simulink model "RobotX_ss_acousticsSingle_Dock_LB_1024"  (R2014a)
settings: Solver=FixedStepDiscrete  StartTime=0.0  StopTime=inf  FixedStep=.25  RelTol=1e-3
undefined symbols (not defined in the file): Com1, Com2, Com3, Com4, DiscIntNeverNeededParam, standard
libraries: xpcseriallib x42, simulink x16, slrtlib x7, dspmtrx3 x2, speedgoatlib x2, speedgoatlib_IO102 x1
(part 3 of 6)

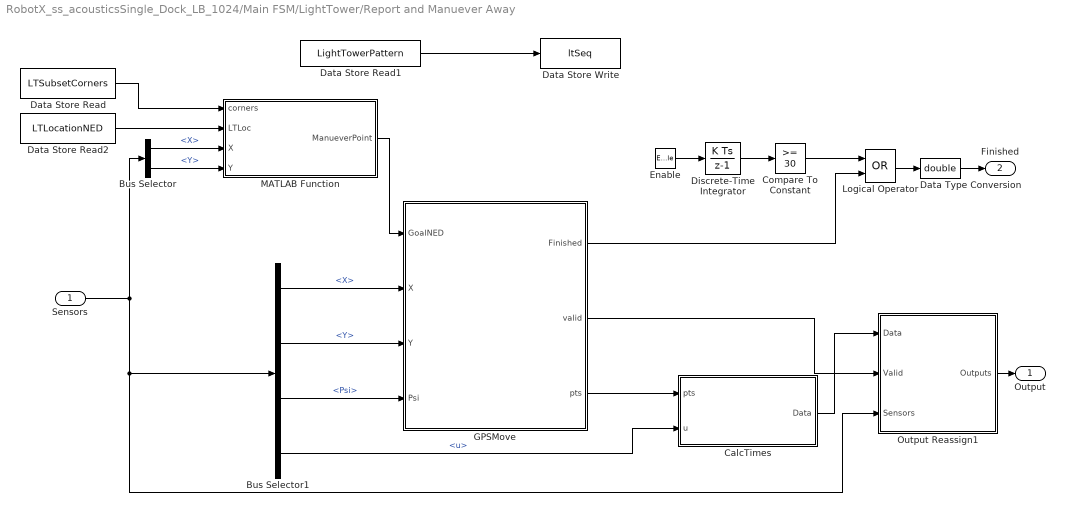
== system RobotX_ss_acousticsSingle_Dock_LB_1024/Main FSM/LightTower/Report and Manuever Away ==
  Sensors : Inport
  Enable : EnablePort  ShowOutputPort=on
  Bus Selector : BusSelector  OutputSignals=Navigation Message.Pose.X,Navigation Message.Pose.Y
  Bus Selector1 : BusSelector  OutputSignals=Navigation Message.Pose.X,Navigation Message.Pose.Y,Navigation Message.Pose.Psi,Navigation Message.Velocity.u
  CalcTimes : MATLAB Function  TreatAsAtomicUnit=on
  Compare To Constant : simulink/Logic and Bit Operations/Compare To Constant  relop=>=  const=30  OutDataTypeStr=boolean
  Data Store Read : DataStoreRead  DataStoreName=LTSubsetCorners
  Data Store Read1 : DataStoreRead  DialogController=Simulink.DDGSource  DataStoreName=LightTowerPattern
  Data Store Read2 : DataStoreRead  DialogController=Simulink.DDGSource  DataStoreName=LTLocationNED
  Data Store Write : DataStoreWrite  DialogController=Simulink.DDGSource  DataStoreName=ltSeq
  Data Type Conversion : DataTypeConversion  OutDataTypeStr=double
  Discrete-Time Integrator : DiscreteIntegrator  SampleTime=-1  ICPrevOutput=DiscIntNeverNeededParam  ICPrevScaledInput=DiscIntNeverNeededParam
  GPSMove : MATLAB Function  TreatAsAtomicUnit=on
  Logical Operator : Logic  Operator=OR  AllPortsSameDT=off  OutDataTypeStr=boolean
  MATLAB Function : MATLAB Function  TreatAsAtomicUnit=on
  Output Reassign1 : Subsystem
  Output : Outport
  Finished : Outport  Port=2
  wires:
  Output Reassign1/1(Outputs) -> Output/1
  Data Store Read/1 -> MATLAB Function/1(corners)
  Sensors/1 -> Bus Selector/1, Output Reassign1/3(Sensors), Bus Selector1/1
  Bus Selector/1 -> MATLAB Function/3(X)  "<X>"
  Bus Selector/2 -> MATLAB Function/4(Y)  "<Y>"
  GPSMove/1(Finished) -> Logical Operator/2
  GPSMove/3(pts) -> CalcTimes/1(pts)
  Bus Selector1/1 -> GPSMove/2(X)  "<X>"
  Bus Selector1/2 -> GPSMove/3(Y)  "<Y>"
  Bus Selector1/3 -> GPSMove/4(Psi)  "<Psi>"
  Bus Selector1/4 -> CalcTimes/2(u)  "<u>"
  CalcTimes/1(Data) -> Output Reassign1/1(Data)
  GPSMove/2(valid) -> Output Reassign1/2(Valid)
  MATLAB Function/1(ManueverPoint) -> GPSMove/1(GoalNED)
  Data Store Read1/1 -> Data Store Write/1
  Data Store Read2/1 -> MATLAB Function/2(LTLoc)
  Discrete-Time Integrator/1 -> Compare To Constant/1
  Enable/1 -> Discrete-Time Integrator/1
  Compare To Constant/1 -> Logical Operator/1
  Logical Operator/1 -> Data Type Conversion/1
  Data Type Conversion/1 -> Finished/1

== system RobotX_ss_acousticsSingle_Dock_LB_1024/Main FSM/LightTower/Sweep Field ==
  Sensors : Inport
  Enable : EnablePort  ShowOutputPort=on
  Bus Creator : BusCreator  Inputs=2
  Bus Selector : BusSelector  OutputSignals=Drive to Point Fin,Spin & Listen Fin
  Compare To Constant : simulink/Logic and Bit Operations/Compare To Constant  relop=>=  const=30  OutDataTypeStr=boolean
  Data Type Conversion : DataTypeConversion  OutDataTypeStr=double
  Discrete-Time Integrator : DiscreteIntegrator  SampleTime=-1  ICPrevOutput=DiscIntNeverNeededParam  ICPrevScaledInput=DiscIntNeverNeededParam
  Drive to Point : Subsystem
  Logical Operator : Logic  Operator=OR  Inputs=3  AllPortsSameDT=off  OutDataTypeStr=boolean
  Multiport Switch : MultiPortSwitch  Inputs=2
  "Spin, Listen, and Point" : Subsystem
  Sweep Field Enabler : MATLAB Function  TreatAsAtomicUnit=on
  Task Option : Subsystem
  Unit Delay : UnitDelay  SampleTime=-1
  Outputs : Outport
  Finished : Outport  Port=2
  wires:
  Drive to Point/1(Outputs) -> Multiport Switch/2
  "Spin, Listen, and Point"/1(Outputs) -> Multiport Switch/3
  Multiport Switch/1 -> Outputs/1
  Data Type Conversion/1 -> Finished/1
  Sensors/1 -> "Spin, Listen, and Point"/1(Sensors), Drive to Point/1(Sensors)
  Task Option/1(Option) -> Sweep Field Enabler/1(Sweep)
  "Spin, Listen, and Point"/2(Finished) -> Bus Creator/2  "Spin & Listen Fin"
  Sweep Field Enabler/2(drivePointEn) -> Drive to Point/Enable
  Sweep Field Enabler/1(taskSelector) -> Multiport Switch/1
  Sweep Field Enabler/3(spinListenEn) -> "Spin, Listen, and Point"/Enable
  Drive to Point/2(Finished) -> Bus Creator/1  "Drive to Point Fin"
  Bus Creator/1 -> Unit Delay/1
  "Spin, Listen, and Point"/3(Found LT) -> Logical Operator/2
  Unit Delay/1 -> Bus Selector/1
  Bus Selector/1 -> Sweep Field Enabler/2(drivePointFin)  "<Drive to Point Fin>"
  Bus Selector/2 -> Sweep Field Enabler/3(spinFin)  "<Spin & Listen Fin>"
  Drive to Point/3(Found LT) -> Logical Operator/1
  Logical Operator/1 -> Data Type Conversion/1
  Discrete-Time Integrator/1 -> Compare To Constant/1
  Enable/1 -> Discrete-Time Integrator/1
  Compare To Constant/1 -> Logical Operator/3

== system RobotX_ss_acousticsSingle_Dock_LB_1024/Main FSM/LightTower/Turn For Approach1  ==
  note: Signal
  Sensors : Inport
  Enable : EnablePort  ShowOutputPort=on
  Bus Selector : BusSelector  OutputSignals=Navigation Message.Pose.X,Navigation Message.Pose.Y
  Compare To Constant : simulink/Logic and Bit Operations/Compare To Constant  relop=>=  const=30  OutDataTypeStr=boolean
  Data Type Conversion : DataTypeConversion  OutDataTypeStr=double
  Discrete-Time Integrator : DiscreteIntegrator  SampleTime=-1  ICPrevOutput=DiscIntNeverNeededParam  ICPrevScaledInput=DiscIntNeverNeededParam
  LTLoc : DataStoreRead  DialogController=Simulink.DDGSource  DataStoreName=LTLocationNED
  MATLAB1 Function : MATLAB Function  TreatAsAtomicUnit=on
  Output Heirarchy : Subsystem
  Outputs : Outport
  Finished : Outport  Port=2
  wires:
  Discrete-Time Integrator/1 -> Compare To Constant/1
  Enable/1 -> Discrete-Time Integrator/1
  Compare To Constant/1 -> Data Type Conversion/1
  Data Type Conversion/1 -> Finished/1
  Sensors/1 -> Bus Selector/1, Output Heirarchy/2(Sensors)
  MATLAB1 Function/1(Data) -> Output Heirarchy/1(Data)
  Output Heirarchy/1(Outputs) -> Outputs/1
  Bus Selector/2 -> MATLAB1 Function/3(Y)  "<Y>"
  Bus Selector/1 -> MATLAB1 Function/2(X)  "<X>"
  LTLoc/1 -> MATLAB1 Function/1(LTLoc)

== system RobotX_ss_acousticsSingle_Dock_LB_1024/Main FSM/LightTower/Turn For Sweep ==
  note: Signal
  Sensors : Inport
  Enable : EnablePort  ShowOutputPort=on
  Bus Selector : BusSelector  OutputSignals=Navigation Message.Pose.X,Navigation Message.Pose.Y
  Compare To Constant : simulink/Logic and Bit Operations/Compare To Constant  relop=>=  const=30  OutDataTypeStr=boolean
  Data Store Read : DataStoreRead  DataStoreName=ltGPS
  Data Store Read1 : DataStoreRead  DataStoreName=NED_origin
  Data Type Conversion : DataTypeConversion  OutDataTypeStr=double
  Discrete-Time Integrator : DiscreteIntegrator  SampleTime=-1  ICPrevOutput=DiscIntNeverNeededParam  ICPrevScaledInput=DiscIntNeverNeededParam
  LLA to NED : MATLAB Function  TreatAsAtomicUnit=on
  MATLAB Function : MATLAB Function  TreatAsAtomicUnit=on
  Output Heirarchy : Subsystem
  Outputs : Outport
  Finished : Outport  Port=2
  wires:
  Discrete-Time Integrator/1 -> Compare To Constant/1
  Enable/1 -> Discrete-Time Integrator/1
  Compare To Constant/1 -> Data Type Conversion/1
  Data Type Conversion/1 -> Finished/1
  Sensors/1 -> Bus Selector/1, Output Heirarchy/2(Sensors)
  MATLAB Function/1(Data) -> Output Heirarchy/1(Data)
  Output Heirarchy/1(Outputs) -> Outputs/1
  Bus Selector/2 -> MATLAB Function/3(Y)  "<Y>"
  Bus Selector/1 -> MATLAB Function/2(X)  "<X>"
  Data Store Read/1 -> LLA to NED/1(GoalLLA)
  Data Store Read1/1 -> LLA to NED/2(NED_origin)
  LLA to NED/1(GoalNED) -> MATLAB Function/1(ltPTS)

== system RobotX_ss_acousticsSingle_Dock_LB_1024/Main FSM/LightTower/Wait for Sequence ==
  Sensors : Inport
  Enable : EnablePort  ShowOutputPort=on
  Bus Selector1 : BusSelector  OutputSignals=Lidar Data Input.Color data.Color
  Data Store Read : DataStoreRead  DataStoreName=holdPose
  Data Store Write : DataStoreWrite  DataStoreName=LightTowerPattern
  Discrete-Time Integrator : DiscreteIntegrator  SampleTime=-1  ICPrevOutput=DiscIntNeverNeededParam  ICPrevScaledInput=DiscIntNeverNeededParam
  MATLAB Function : MATLAB Function  TreatAsAtomicUnit=on
  MATLAB Function1 : MATLAB Function  TreatAsAtomicUnit=on
  Output Reassign1 : Subsystem
  Output : Outport
  Finished : Outport  Port=2
  wires:
  Sensors/1 -> Bus Selector1/1, Output Reassign1/2(Sensors)
  Output Reassign1/1(Outputs) -> Output/1
  MATLAB Function/1(Data) -> Output Reassign1/1(Data)
  MATLAB Function1/2(Pattern) -> Data Store Write/1
  Bus Selector1/1 -> MATLAB Function1/2(visionData)  "<Color>"
  Enable/1 -> Discrete-Time Integrator/1
  Discrete-Time Integrator/1 -> MATLAB Function1/1(time)
  MATLAB Function1/1(Finished) -> Finished/1
  Data Store Read/1 -> MATLAB Function/1(holdPose)

== system RobotX_ss_acousticsSingle_Dock_LB_1024/Main FSM/RCHold/Direct Control ==
  Sensors : Inport
  Acoustic Active : Constant  Value=0
  Bus Creator2 : BusCreator  Inputs=3
  Bus Creator3 : BusCreator  Inputs=3
  Bus Creator4 : BusCreator  Inputs=2
  Constant : Constant
  Constant1 : Constant  Value=2
  Constant2 : Constant  Value=zeros(24,1)
  Lidar Mode : Constant  Value=3
  Outputs : Outport
  wires:
  Sensors/1 -> Bus Creator4/2  "Sensors"
  Bus Creator4/1 -> Outputs/1  "Output Signals"
  Bus Creator2/1 -> Bus Creator3/1  "Navigation Outputs"
  Acoustic Active/1 -> Bus Creator3/2  "Acoustic Active"
  Lidar Mode/1 -> Bus Creator3/3  "Lidar Mode"
  Bus Creator3/1 -> Bus Creator4/1  "Outputs"
  Constant/1 -> Bus Creator2/1  "Valid"
  Constant1/1 -> Bus Creator2/2  "Control Mode"
  Constant2/1 -> Bus Creator2/3  "Data"

== system RobotX_ss_acousticsSingle_Dock_LB_1024/Main FSM/Start//Speedgate/Aim ==
  note: Signal
  Sensors : Inport
  Enable : EnablePort  ShowOutputPort=on
  Compare To Constant : simulink/Logic and Bit Operations/Compare To Constant  relop=>=  const=30  OutDataTypeStr=boolean
  Data Store Read : DataStoreRead  DataStoreName=ssHeldHeading
  Data Store Read1 : DataStoreRead  Commented=on  DataStoreName=startGPS
  Data Store Read2 : DataStoreRead  Commented=on  DataStoreName=NED_origin
  Data Store Read3 : DataStoreRead  DataStoreName=startNED
  Data Type Conversion : DataTypeConversion  OutDataTypeStr=double
  Discrete-Time Integrator : DiscreteIntegrator  SampleTime=-1  ICPrevOutput=DiscIntNeverNeededParam  ICPrevScaledInput=DiscIntNeverNeededParam
  LLA to NED : MATLAB Function  Commented=on  TreatAsAtomicUnit=on
  MATLAB Function : MATLAB Function  TreatAsAtomicUnit=on
  Output Heirarchy : Subsystem
  Outputs : Outport
  Finished : Outport  Port=2
  wires:
  Discrete-Time Integrator/1 -> Compare To Constant/1
  Enable/1 -> Discrete-Time Integrator/1
  Compare To Constant/1 -> Data Type Conversion/1
  Data Type Conversion/1 -> Finished/1
  Sensors/1 -> Output Heirarchy/2(Sensors)
  MATLAB Function/1(Data) -> Output Heirarchy/1(Data)
  Output Heirarchy/1(Outputs) -> Outputs/1
  Data Store Read/1 -> MATLAB Function/1(ssHeldHeading)
  LLA to NED/1(GoalNED) -> ?
  Data Store Read2/1 -> LLA to NED/2(NED_origin)
  Data Store Read1/1 -> LLA to NED/1(LLA)
  Data Store Read3/1 -> MATLAB Function/2(ssGateNED)

== system RobotX_ss_acousticsSingle_Dock_LB_1024/Main FSM/Start//Speedgate/Dead Reckon ==
  note: Through Gate
  Sensors : Inport
  Enable : EnablePort
  Bus Selector : BusSelector  OutputSignals=Navigation Message.Pose.X,Navigation Message.Pose.Y,Navigation Message.Velocity.u
  Calculate Times : MATLAB Function  TreatAsAtomicUnit=on
  Data Store Read : DataStoreRead  DataStoreName=ssHeldHeading
  Gate : MATLAB Function  TreatAsAtomicUnit=on
  Output Reassign : Subsystem
  sglength : Constant  Value=15
  Outputs : Outport
  Finished : Outport  Port=2
  wires:
  Output Reassign/1(Outputs) -> Outputs/1
  Gate/1(Finished) -> Finished/1
  Sensors/1 -> Output Reassign/3(Sensors), Bus Selector/1
  Bus Selector/2 -> Gate/4(Y)  "<Y>"
  Bus Selector/1 -> Gate/3(X)  "<X>"
  Bus Selector/3 -> Calculate Times/2(u)  "<u>"
  Gate/3(pts) -> Calculate Times/1(pts)
  Calculate Times/1(Data) -> Output Reassign/2(Data)
  Gate/2(Valid) -> Output Reassign/1(Vaild)
  Data Store Read/1 -> Gate/2(ssHeldHeading)
  sglength/1 -> Gate/1(sglength)

== system RobotX_ss_acousticsSingle_Dock_LB_1024/Main FSM/Start//Speedgate/GPS Move ==
  Sensors : Inport
  Enable : EnablePort
  Bus Selector : BusSelector  OutputSignals=Navigation Message.Pose.X,Navigation Message.Pose.Y,Navigation Message.Pose.Psi,Navigation Message.Velocity.u
  CalcTimes : MATLAB Function  TreatAsAtomicUnit=on
  Data Store Read1 : DataStoreRead  Commented=on  DataStoreName=startGPS
  Data Store Read2 : DataStoreRead  Commented=on  DataStoreName=NED_origin
  Data Store Read3 : DataStoreRead  DataStoreName=startNED
  GPSMove : MATLAB Function  TreatAsAtomicUnit=on
  LLA to NED : MATLAB Function  Commented=on  TreatAsAtomicUnit=on
  Output Reassign : Subsystem
  Outputs : Outport
  Finished : Outport  Port=2
  wires:
  GPSMove/3(pts) -> CalcTimes/1(pts)
  Sensors/1 -> Output Reassign/3(Sensors), Bus Selector/1
  Bus Selector/1 -> GPSMove/2(X)  "<X>"
  Bus Selector/2 -> GPSMove/3(Y)  "<Y>"
  Bus Selector/3 -> GPSMove/4(Psi)  "<Psi>"
  Bus Selector/4 -> CalcTimes/2(u)  "<u>"
  GPSMove/1(Finished) -> Finished/1
  Output Reassign/1(Outputs) -> Outputs/1
  CalcTimes/1(Data) -> Output Reassign/2(Data)
  GPSMove/2(valid) -> Output Reassign/1(Vaild)
  LLA to NED/1(GoalNED) -> ?
  Data Store Read3/1 -> GPSMove/1(GoalNED)
  Data Store Read2/1 -> LLA to NED/2(NED_origin)
  Data Store Read1/1 -> LLA to NED/1(LLA)

== system RobotX_ss_acousticsSingle_Dock_LB_1024/Main FSM/Termination/Output Reassign ==
  Vaild : Inport
  Data : Inport  Port=2
  Sensors : Inport  Port=3
  Acoustic Active : Constant  Value=0
  Bus Creator2 : BusCreator  Inputs=3
  Bus Creator3 : BusCreator  Inputs=3
  Bus Creator5 : BusCreator  Inputs=2
  Constant3 : Constant  Value=0
  Lidar Mode : Constant  Value=0
  Outputs : Outport
  wires:
  Sensors/1 -> Bus Creator5/2  "Sensors"
  Bus Creator5/1 -> Outputs/1  "Output Signals"
  Vaild/1 -> Bus Creator2/1  "Valid"
  Constant3/1 -> Bus Creator2/2  "Control Mode"
  Data/1 -> Bus Creator2/3  "Data"
  Bus Creator2/1 -> Bus Creator3/1  "Navigation Outputs"
  Acoustic Active/1 -> Bus Creator3/2  "Acoustic Active"
  Lidar Mode/1 -> Bus Creator3/3  "Lidar Mode"
  Bus Creator3/1 -> Bus Creator5/1  "Outputs"

== system RobotX_ss_acousticsSingle_Dock_LB_1024/Sensors/1020 Comms/ Raspberry Pi LCM (Acoustic) ==
  LCM Input : Inport
  ASCII Decode 6 : xpcseriallib/ASCII Decode   format=Deploy:%1u, Elapsed:%g, Bearing1:%g Bearing2:%g \r\n  nvars=4  vartypes={}
  Bus Creator : BusCreator  Inputs=2
  Bus Creator1 : BusCreator  Inputs=3
  FIFO ASCII read 1 : xpcseriallib/FIFO ASCII read   header={'Deploy:'}  term=[13 10]  hold=Zero output if no new data  enable=off  maxsize=1024  outputtype=8 bit uint null terminated  sampletime=-1
  LCM Output : Outport
  wires:
  LCM Input/1 -> FIFO ASCII read 1/1
  FIFO ASCII read 1/1 -> ASCII Decode 6/1
  ASCII Decode 6/3 -> Bus Creator/1  "Horizontal Bearing"
  ASCII Decode 6/4 -> Bus Creator/2  "Vertical Bearing"
  Bus Creator/1 -> Bus Creator1/3  "Bearings"
  ASCII Decode 6/2 -> Bus Creator1/2  "Elapsed Time"
  ASCII Decode 6/1 -> Bus Creator1/1  "Deployed"
  Bus Creator1/1 -> LCM Output/1  "Acoustic Message"

== system RobotX_ss_acousticsSingle_Dock_LB_1024/Sensors/1020 Comms/ Raspberry Pi LCM (Navigation and Acoustics) ==
  LCM Input : Inport
  ASCII Decode 6 : xpcseriallib/ASCII Decode   format=P1:%f P2:%f P3:%f V1:%f V2:%f V3:%f E1:%f E2:%f E3:%f Pt1:%f Pt2:%f St1:%f St2:%f Start:%f Elapsed:%f RC:%d Deploy:%u, Elapsed:%g, Bearing1:%g Bearing2:%g \r\n  nvars=22  vartypes={}
  Bus Creator{,5..7} (4 alike) : BusCreator  Inputs=2
  Bus Creator{1..3,8} (4 alike) : BusCreator  Inputs=3
  Bus Creator4 : BusCreator  Inputs=9
  Data Type Conversion : DataTypeConversion  OutDataTypeStr=double
  FIFO ASCII read 1 : xpcseriallib/FIFO ASCII read   header={'P1:'}  term=[13 10]  hold=Zero output if no new data  enable=off  maxsize=2048  outputtype=8 bit uint null terminated  sampletime=-1
  Navigation LCM : Outport
  Acoustic LCM : Outport  Port=2
  wires:
  LCM Input/1 -> FIFO ASCII read 1/1
  FIFO ASCII read 1/1 -> ASCII Decode 6/1
  Bus Creator4/1 -> Navigation LCM/1  "Navigation Message"
  ASCII Decode 6/1 -> Bus Creator1/1  "X"
  ASCII Decode 6/2 -> Bus Creator1/2  "Y"
  ASCII Decode 6/3 -> Bus Creator1/3  "Psi"
  Bus Creator1/1 -> Bus Creator4/1  "Pose"
  ASCII Decode 6/4 -> Bus Creator2/1  "u"
  ASCII Decode 6/5 -> Bus Creator2/2  "v"
  Bus Creator2/1 -> Bus Creator4/2  "Velocity"
  ASCII Decode 6/7 -> Bus Creator3/1  "Roll"
  ASCII Decode 6/8 -> Bus Creator3/2  "Pitch"
  ASCII Decode 6/9 -> Bus Creator3/3  "Yaw"
  Bus Creator3/1 -> Bus Creator4/3  "Euler"
  Bus Creator5/1 -> Bus Creator4/5  "Port"
  Bus Creator6/1 -> Bus Creator4/6  "Stbd"
  ASCII Decode 6/14 -> Bus Creator6/1  "StThrust"
  ASCII Decode 6/15 -> Bus Creator6/2  "StAzimuth"
  ASCII Decode 6/12 -> Bus Creator5/1  "PtThrust"
  ASCII Decode 6/13 -> Bus Creator5/2  "PtAzimuth"
  ASCII Decode 6/16 -> Bus Creator4/7  "Start"
  ASCII Decode 6/17 -> Bus Creator4/8  "Elapsed"
  ASCII Decode 6/18 -> Data Type Conversion/1  "On/Off/RC/Auto"
  Data Type Conversion/1 -> Bus Creator4/9  "On/Off/RC/Auto"
  ASCII Decode 6/6 -> Bus Creator2/3  "r"
  ASCII Decode 6/10 -> Bus Creator7/1  "Lat"
  ASCII Decode 6/11 -> Bus Creator7/2  "Long"
  Bus Creator7/1 -> Bus Creator4/4  "GPS (LLA)"
  ASCII Decode 6/21 -> Bus Creator/1  "Horizontal Bearing"
  ASCII Decode 6/22 -> Bus Creator/2  "Vertical Bearing"
  Bus Creator/1 -> Bus Creator8/3  "Bearings"
  ASCII Decode 6/20 -> Bus Creator8/2  "Elapsed Time"
  ASCII Decode 6/19 -> Bus Creator8/1  "Deployed"
  Bus Creator8/1 -> Acoustic LCM/1  "Acoustic Message"

== system RobotX_ss_acousticsSingle_Dock_LB_1024/Sensors/1020 Comms/ Raspberry Pi LCM (Navigation) ==
  LCM Input : Inport
  ASCII Decode 6 : xpcseriallib/ASCII Decode   format=P1:%f P2:%f P3:%f V1:%f V2:%f V3:%f E1:%f E2:%f E3:%f Lat:%f Long:%f Pt1:%f Pt2:%f St1:%f St2:%f Start:%f Elapsed:%f RC:%d Deploy:%u Elapsed:%f Bearing1:%f Bearing2:%f Range:%f X_Pos:%f Y_Pos:%f \r\n  nvars=25  vartypes={}
  Bus Creator1 : BusCreator  Inputs=3
  Bus Creator2 : BusCreator  Inputs=3
  Bus Creator3 : BusCreator  Inputs=3
  Bus Creator4 : BusCreator  Inputs=9
  Bus Creator5 : BusCreator  Inputs=2
  Bus Creator6 : BusCreator  Inputs=2
  Bus Creator7 : BusCreator  Inputs=2
  Bus Creator8 : BusCreator  Inputs=7
  Data Type Conversion : DataTypeConversion  OutDataTypeStr=double
  FIFO ASCII read 1 : xpcseriallib/FIFO ASCII read   header={'P1:'}  term=[13 10]  hold=Zero output if no new data  enable=off  maxsize=2000  outputtype=8 bit uint null terminated  sampletime=-1
  LCM Output : Outport
  Acou LCM : Outport  Port=2
  wires:
  LCM Input/1 -> FIFO ASCII read 1/1
  FIFO ASCII read 1/1 -> ASCII Decode 6/1
  Bus Creator4/1 -> LCM Output/1  "Navigation Message"
  ASCII Decode 6/1 -> Bus Creator1/1  "X"
  ASCII Decode 6/2 -> Bus Creator1/2  "Y"
  ASCII Decode 6/3 -> Bus Creator1/3  "Psi"
  Bus Creator1/1 -> Bus Creator4/1  "Pose"
  ASCII Decode 6/4 -> Bus Creator2/1  "u"
  ASCII Decode 6/5 -> Bus Creator2/2  "v"
  Bus Creator2/1 -> Bus Creator4/2  "Velocity"
  ASCII Decode 6/7 -> Bus Creator3/1  "Roll"
  ASCII Decode 6/8 -> Bus Creator3/2  "Pitch"
  ASCII Decode 6/9 -> Bus Creator3/3  "Yaw"
  Bus Creator3/1 -> Bus Creator4/3  "Euler"
  Bus Creator5/1 -> Bus Creator4/5  "Port"
  Bus Creator6/1 -> Bus Creator4/6  "Stbd"
  ASCII Decode 6/14 -> Bus Creator6/1  "StThrust"
  ASCII Decode 6/15 -> Bus Creator6/2  "StAzimuth"
  ASCII Decode 6/12 -> Bus Creator5/1  "PtThrust"
  ASCII Decode 6/13 -> Bus Creator5/2  "PtAzimuth"
  ASCII Decode 6/16 -> Bus Creator4/7  "Start"
  ASCII Decode 6/17 -> Bus Creator4/8  "Elapsed"
  ASCII Decode 6/18 -> Data Type Conversion/1  "On/Off/RC/Auto"
  Data Type Conversion/1 -> Bus Creator4/9  "On/Off/RC/Auto"
  ASCII Decode 6/6 -> Bus Creator2/3  "r"
  ASCII Decode 6/10 -> Bus Creator7/1  "Lat"
  ASCII Decode 6/11 -> Bus Creator7/2  "Long"
  Bus Creator7/1 -> Bus Creator4/4  "GPS (LLA)"
  ASCII Decode 6/19 -> Bus Creator8/1  "Deployed"
  ASCII Decode 6/20 -> Bus Creator8/2  "Elapsed Time"
  ASCII Decode 6/21 -> Bus Creator8/3  "Horizontal Bearing"
  ASCII Decode 6/22 -> Bus Creator8/4  "Vertical Bearing"
  ASCII Decode 6/23 -> Bus Creator8/5  "Range"
  ASCII Decode 6/24 -> Bus Creator8/6  "X Pos"
  ASCII Decode 6/25 -> Bus Creator8/7  "Y Pos"
  Bus Creator8/1 -> Acou LCM/1

== system RobotX_ss_acousticsSingle_Dock_LB_1024/Sensors/1020 Comms/Acoustic LCM ==
  LCM Input : Inport
  Bus Creator : BusCreator  Inputs=2
  Bus Creator1 : BusCreator
  Bus Creator2 : BusCreator  Inputs=3
  Bus Selector : BusSelector  OutputSignals=Deployed,Elapsed Time,Horizontal Bearing,Vertical Bearing,Range,X Pos,Y Pos
  LCM Output : Outport
  wires:
  Bus Selector/3 -> Bus Creator/1  "<Horizontal Bearing>"
  Bus Selector/4 -> Bus Creator/2  "<Vertical Bearing>"
  Bus Creator/1 -> Bus Creator1/3  "Bearings"
  Bus Selector/2 -> Bus Creator1/2  "<Elapsed Time>"
  Bus Selector/1 -> Bus Creator1/1  "<Deployed>"
  Bus Creator1/1 -> LCM Output/1  "Acoustic Message"
  LCM Input/1 -> Bus Selector/1
  Bus Selector/5 -> Bus Creator2/1  "<Range>"
  Bus Selector/6 -> Bus Creator2/2  "<X Pos>"
  Bus Selector/7 -> Bus Creator2/3  "<Y Pos>"
  Bus Creator2/1 -> Bus Creator1/4  "Pose Estimate"

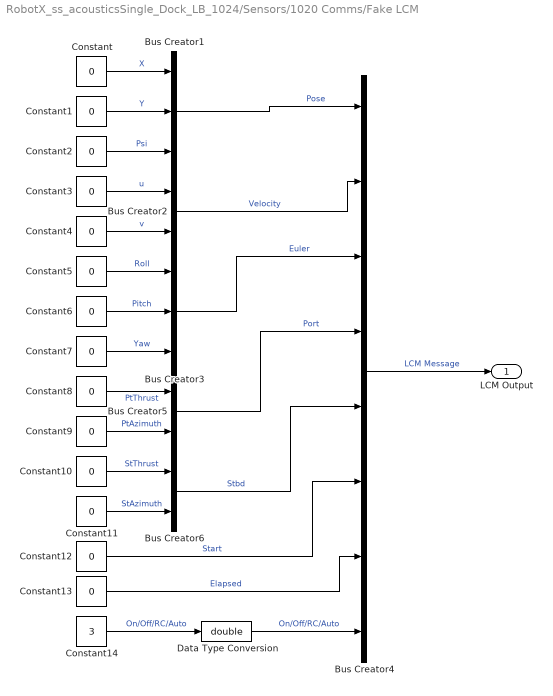
== system RobotX_ss_acousticsSingle_Dock_LB_1024/Sensors/1020 Comms/Fake LCM ==
  Bus Creator1 : BusCreator  Inputs=3
  Bus Creator2 : BusCreator  Inputs=2
  Bus Creator3 : BusCreator  Inputs=3
  Bus Creator4 : BusCreator  Inputs=8
  Bus Creator5 : BusCreator  Inputs=2
  Bus Creator6 : BusCreator  Inputs=2
  Constant{,1..13} (14 alike) : Constant  Value=0
  Constant14 : Constant  Value=3
  Data Type Conversion : DataTypeConversion  OutDataTypeStr=double
  LCM Output : Outport
  wires:
  Bus Creator4/1 -> LCM Output/1  "LCM Message"
  Constant/1 -> Bus Creator1/1  "X"
  Constant1/1 -> Bus Creator1/2  "Y"
  Constant2/1 -> Bus Creator1/3  "Psi"
  Bus Creator1/1 -> Bus Creator4/1  "Pose"
  Constant3/1 -> Bus Creator2/1  "u"
  Constant4/1 -> Bus Creator2/2  "v"
  Bus Creator2/1 -> Bus Creator4/2  "Velocity"
  Constant5/1 -> Bus Creator3/1  "Roll"
  Constant6/1 -> Bus Creator3/2  "Pitch"
  Constant7/1 -> Bus Creator3/3  "Yaw"
  Bus Creator3/1 -> Bus Creator4/3  "Euler"
  Bus Creator5/1 -> Bus Creator4/4  "Port"
  Bus Creator6/1 -> Bus Creator4/5  "Stbd"
  Constant10/1 -> Bus Creator6/1  "StThrust"
  Constant11/1 -> Bus Creator6/2  "StAzimuth"
  Constant8/1 -> Bus Creator5/1  "PtThrust"
  Constant9/1 -> Bus Creator5/2  "PtAzimuth"
  Constant12/1 -> Bus Creator4/6  "Start"
  Constant13/1 -> Bus Creator4/7  "Elapsed"
  Constant14/1 -> Data Type Conversion/1  "On/Off/RC/Auto"
  Data Type Conversion/1 -> Bus Creator4/8  "On/Off/RC/Auto"

== system RobotX_ss_acousticsSingle_Dock_LB_1024/Sensors/1020 Comms/LIDAR Panda ==
  LIDAR Panda In : Inport
  ASCII Decode 2 : xpcseriallib/ASCII Decode   format=A:%d B:%d C:%d E:%d F:%d G:%d H:%d I:%d J:%d K:%d L:%d M:%d N:%d O:%d P:%d Q:%d R:%d S:%d T:%d U:%d V:%d W:%d X:%d C1:%d C2:%d C3:%d C4:%d P1:%f P2:%f P3:%f P4:%f I1:%d I2:%d I3:%d I4:%d \r\n  nvars=36  vartypes={}
  Bus Creator1 : BusCreator  Inputs=2
  Bus Creator2 : BusCreator  Inputs=3
  Bus Creator3 : BusCreator  Inputs=2
  Data Type Conversion{,1..3} (4 alike) : DataTypeConversion  OutDataTypeStr=double
  "FIFO ASCII read " : xpcseriallib/FIFO ASCII read   header={'A:'}  term=[13 10]  hold=Zero output if no new data  enable=off  maxsize=1024  outputtype=8 bit uint null terminated  sampletime=-1
  Mux : Mux  Inputs=12
  Mux1 : Mux
  Mux2 : Mux  Inputs=12
  Mux3 : Mux
  Mux4 : Mux
  LIDAR Panda Out : Outport
  wires:
  LIDAR Panda In/1 -> "FIFO ASCII read "/1
  "FIFO ASCII read "/1 -> ASCII Decode 2/1
  ASCII Decode 2/3 -> Mux/3  "Distance"
  ASCII Decode 2/2 -> Mux/2  "Color ID"
  ASCII Decode 2/4 -> Mux/4  "Angle"
  ASCII Decode 2/1 -> Mux/1  "Probability"
  ASCII Decode 2/7 -> Mux/7
  ASCII Decode 2/10 -> Mux/10
  ASCII Decode 2/11 -> Mux/11
  ASCII Decode 2/6 -> Mux/6
  ASCII Decode 2/8 -> Mux/8
  ASCII Decode 2/9 -> Mux/9
  ASCII Decode 2/12 -> Mux/12
  ASCII Decode 2/5 -> Mux/5
  ASCII Decode 2/13 -> Mux2/1
  ASCII Decode 2/15 -> Mux2/3
  ASCII Decode 2/22 -> Mux2/10
  ASCII Decode 2/23 -> Mux2/11
  ASCII Decode 2/17 -> Mux2/5
  ASCII Decode 2/18 -> Mux2/6
  ASCII Decode 2/14 -> Mux2/2
  ASCII Decode 2/24 -> Mux2/12
  ASCII Decode 2/20 -> Mux2/8
  ASCII Decode 2/19 -> Mux2/7
  ASCII Decode 2/21 -> Mux2/9
  ASCII Decode 2/16 -> Mux2/4
  ASCII Decode 2/25 -> Mux1/1
  ASCII Decode 2/28 -> Mux1/4
  ASCII Decode 2/26 -> Mux1/2
  ASCII Decode 2/27 -> Mux1/3
  ASCII Decode 2/30 -> Mux3/2
  ASCII Decode 2/31 -> Mux3/3
  ASCII Decode 2/32 -> Mux3/4
  ASCII Decode 2/29 -> Mux3/1
  ASCII Decode 2/36 -> Mux4/4
  ASCII Decode 2/34 -> Mux4/2
  ASCII Decode 2/35 -> Mux4/3
  ASCII Decode 2/33 -> Mux4/1
  Mux/1 -> Data Type Conversion/1  "Distances"
  Mux2/1 -> Data Type Conversion1/1  "Angles"
  Mux1/1 -> Data Type Conversion2/1  "Color"
  Mux3/1 -> Bus Creator2/2  "Probability"
  Mux4/1 -> Data Type Conversion3/1  "idx"
  Bus Creator1/1 -> Bus Creator3/1  "Landmarks"
  Bus Creator2/1 -> Bus Creator3/2  "Color data"
  Bus Creator3/1 -> LIDAR Panda Out/1
  Data Type Conversion/1 -> Bus Creator1/1  "Distances"
  Data Type Conversion1/1 -> Bus Creator1/2  "Angles"
  Data Type Conversion2/1 -> Bus Creator2/1  "Color"
  Data Type Conversion3/1 -> Bus Creator2/3  "Color"

== system RobotX_ss_acousticsSingle_Dock_LB_1024/Sensors/1020 Comms/Subsystem ==
  Bus Creator : BusCreator  Inputs=3
  Bus Creator1 : BusCreator  Inputs=2
  Bus Creator2 : BusCreator  Inputs=2
  Constant : Constant  Value=zeros(12,1)
  Constant1 : Constant  Value=zeros(12,1)
  Constant2 : Constant  Value=zeros(4,1)
  Constant3 : Constant  Value=zeros(4,1)
  Constant4 : Constant  Value=zeros(4,1)
  Fake Panda : Outport
  wires:
  Constant/1 -> Bus Creator1/1  "Distances"
  Constant1/1 -> Bus Creator1/2  "Angles"
  Constant2/1 -> Bus Creator/1  "Color"
  Constant3/1 -> Bus Creator/2  "Probability"
  Constant4/1 -> Bus Creator/3  "idx"
  Bus Creator1/1 -> Bus Creator2/1  "Landmarks"
  Bus Creator/1 -> Bus Creator2/2  "Color data"
  Bus Creator2/1 -> Fake Panda/1  "Lidar Data Input"

== system RobotX_ss_acousticsSingle_Dock_LB_1024/Sensors/1020 Comms/data log ==
  Sensors signal : Inport
  Bus Selector3 : BusSelector  OutputSignals=Navigation Message,Lidar Data Input,Acoustic Message
  Bus to Vector : BusToVector
  Bus to Vector1 : BusToVector
  Bus to Vector2 : BusToVector
  Read : DataStoreRead  DataStoreName=PingPose
  Scope 1 : slrtlib/Displays and Logging/Scope   scopeno=3  scopetype=File  autostart=on  viewmode=Graphical redraw  formatstr='%15.6f'  grid=on  ylimits=[0,0]  nosamples=28800  noprepostsamples=0  interleave=1  triggermode=FreeRun  triggersignal=1  trigsignalfromport=off  triggerlevel=0.0  triggerslope=Either  triggerscope=1  triggersample=0  filename=LM1_<%%%>.dat  mode=Lazy  writesize=5120  autorestart=on  dynamicfilemode=on  maxwritefilesize=512*1024^2
  Scope 2 : slrtlib/Displays and Logging/Scope   scopeno=1  scopetype=File  autostart=on  viewmode=Graphical redraw  formatstr='%15.6f'  grid=on  ylimits=[0,0]  nosamples=28800  noprepostsamples=0  interleave=1  triggermode=FreeRun  triggersignal=1  trigsignalfromport=off  triggerlevel=0.0  triggerslope=Either  triggerscope=1  triggersample=0  filename=NAV1_<%%%>.dat  mode=Lazy  writesize=5120  autorestart=on  dynamicfilemode=on  maxwritefilesize=512*1024^2
  Scope 3 : slrtlib/Displays and Logging/Scope   scopeno=2  scopetype=File  autostart=on  viewmode=Graphical redraw  formatstr='%15.6f'  grid=on  ylimits=[0,0]  nosamples=28800  noprepostsamples=0  interleave=1  triggermode=FreeRun  triggersignal=1  trigsignalfromport=off  triggerlevel=0.0  triggerslope=Either  triggerscope=1  triggersample=0  filename=ACO1_<%%%>.dat  mode=Lazy  writesize=5120  autorestart=on  dynamicfilemode=on  maxwritefilesize=512*1024^2
  Scope 4 : slrtlib/Displays and Logging/Scope   scopeno=4  scopetype=File  autostart=on  viewmode=Graphical redraw  formatstr='%15.6f'  grid=on  ylimits=[0,0]  nosamples=28800  noprepostsamples=0  interleave=1  triggermode=FreeRun  triggersignal=1  trigsignalfromport=off  triggerlevel=0.0  triggerslope=Either  triggerscope=1  triggersample=0  filename=pPos_<%%%>.dat  mode=Lazy  writesize=5120  autorestart=on  dynamicfilemode=on  maxwritefilesize=512*1024^2
  wires:
  Sensors signal/1 -> Bus Selector3/1
  Bus to Vector/1 -> Scope 2/1
  Bus Selector3/1 -> Bus to Vector/1  "<Navigation Message>"
  Bus to Vector1/1 -> Scope 1/1
  Bus to Vector2/1 -> Scope 3/1
  Bus Selector3/3 -> Bus to Vector2/1  "<Acoustic Message>"
  Bus Selector3/2 -> Bus to Vector1/1  "<Lidar Data Input>"
  Read/1 -> Scope 4/1

== system RobotX_ss_acousticsSingle_Dock_LB_1024/Sensors/1024 Comms/ Raspberry Pi LCM (Acoustic) ==
  LCM Input : Inport
  ASCII Decode 6 : xpcseriallib/ASCII Decode   format=Deploy:%1u, Elapsed:%g, Bearing1:%g Bearing2:%g \r\n  nvars=4  vartypes={}
  Bus Creator : BusCreator  Inputs=2
  Bus Creator1 : BusCreator  Inputs=3
  FIFO ASCII read 1 : xpcseriallib/FIFO ASCII read   header={'Deploy:'}  term=[13 10]  hold=Zero output if no new data  enable=off  maxsize=1024  outputtype=8 bit uint null terminated  sampletime=-1
  LCM Output : Outport
  wires:
  LCM Input/1 -> FIFO ASCII read 1/1
  FIFO ASCII read 1/1 -> ASCII Decode 6/1
  ASCII Decode 6/3 -> Bus Creator/1  "Horizontal Bearing"
  ASCII Decode 6/4 -> Bus Creator/2  "Vertical Bearing"
  Bus Creator/1 -> Bus Creator1/3  "Bearings"
  ASCII Decode 6/2 -> Bus Creator1/2  "Elapsed Time"
  ASCII Decode 6/1 -> Bus Creator1/1  "Deployed"
  Bus Creator1/1 -> LCM Output/1  "Acoustic Message"

== matlab function RobotX_ss_acousticsSingle_Dock_LB_1024/Sensors/1024 Comms/Message Selector/HRTLIT Message/MATLAB Function ==
  data: Time input; HRTLat input; HRTLong input; HRTTask input; HRTMode input; LITValid input; asciiHRTLIT output; LITSequence input
function asciiHRTLIT = asciiHRTLITEncoder(Time,HRTLat,HRTLong,HRTTask,HRTMode,LITValid,LITSequence)
% Initialize output message vector as the serial output block expects 128
% character message
asciiHRTLIT = uint8(zeros(1,128));

asciiComma = uint8(',');
asciiDeciPt = uint8('.');
asciiTeamID = uint8('FAUVU,');
asciiMsgEnd = uint8('*');
asciiMsgCRLF = [13 10];

% Convert UTC Time input (hhmmss) into ascii code
asciiTime = uint8(zeros(1,7));
asciiTime(7) = asciiComma;

for timeChar = 1:6
    asciiTime(timeChar) = floor(mod(Time,10^(7-timeChar))/...
        10^(6-timeChar)) + 48;
end

%%%%%%%%%%%%%%%%%%%%%%%%%%%%%%%%%%%%%%%%%%%%%%%%%%%%%%%%%%%%%%%%%%%%
% Heartbeat message
% Convert static strings to ascii code
asciiHRTMsgID = uint8('$RXHRT,');
if HRTLat >= 0
    asciiHRTNS = uint8('N,');
else
    HRTLat = -HRTLat;
    asciiHRTNS = uint8('S,');
end
if HRTLong >= 0
    asciiHRTEW = uint8('E,');
else
    HRTLong = -HRTLong;
    asciiHRTEW = uint8('W,');
end

% Convert latitude (dd.mmmmmm) into ascii code
asciiHRTLat = uint8(zeros(1,10));
asciiHRTLat(10) = asciiComma;
asciiHRTLat(3) = asciiDeciPt;

HRTlatInt = floor(HRTLat);
for latIntChar = 1:2
    asciiHRTLat(latIntChar) = floor(mod(HRTlatInt,10^(3-latIntChar))/...
        10^(2-latIntChar)) + 48;
end

HRTlatDeci = mod(HRTLat,HRTlatInt) * 10^6;
for latDeciChar = 1:6
    asciiHRTLat(latDeciChar+3) = floor(mod(HRTlatDeci,10^(7-latDeciChar))/...
        10^(6-latDeciChar)) + 48;
end

% Convert longitude (ddd.mmmmmm) into ascii code
asciiHRTLong = uint8(zeros(1,11));
asciiHRTLong(11) = asciiComma;
asciiHRTLong(4) = asciiDeciPt;

HRTlongInt = floor(HRTLong);
for longIntChar = 1:3
    asciiHRTLong(longIntChar) = floor(mod(HRTlongInt,10^(4-longIntChar))/...
        10^(3-longIntChar)) + 48;
end

HRTlongDeci = mod(HRTLong,HRTlongInt) * 10^6;
for longDeciChar = 1:6
    asciiHRTLong(longDeciChar+4) = floor(mod(HRTlongDeci,10^(7-longDeciChar))/...
        10^(6-longDeciChar)) + 48;
end

% Convert vehicle mode into ascii (1 = RC, 2 = Auto)

% Auto On 
if HRTMode == 3 
    HRTOpMode = 2;
    asciiHRTMode = [uint8(HRTOpMode+48) asciiComma];
else
    HRTOpMode = 1;
    asciiHRTMode = [uint8(HRTOpMode+48) asciiComma];
end

% Convert vehicle task into ascii
HRTTask = HRTTask - 1; % FSM: Init = 1, SSGate = 2, SEA = 3, Dock = 4, LIT = 5, Obst = 6
if HRTTask ~= 1 || 2 || 3 || 4 || 5
    HRTOpTask = 1;
    asciiHRTTask = [uint8(HRTOpTask+48) asciiMsgEnd];
else
    asciiHRTTask = [uint8(HRTTask+48) asciiMsgEnd];
end

% Concat individual ascii arrays into one array
asciiHRTPreChkSum = cat(2,asciiHRTMsgID,asciiTime,asciiHRTLat,asciiHRTNS,asciiHRTLong,asciiHRTEW,...
    asciiTeamID,asciiHRTMode,asciiHRTTask);

% Calculate the checksum of the message from the '$' to the '*' and convert
% to hex
HRTchkSum = uint8(0);

for chksumChar = 1:(length(asciiHRTPreChkSum)-2)
    HRTchkSum = bitxor(HRTchkSum,asciiHRTPreChkSum(chksumChar+1));
end

% Convert the checksum to ascii
HRTchkSum = dec2hex(HRTchkSum);
asciiHRTChkSum = uint8(zeros(1,length(HRTchkSum))+32);
for i = 1:length(HRTchkSum)
    asciiHRTChkSum(i) = uint8(HRTchkSum(i));
end

% Concat the checksum and the '/r/n' to the end of the message
asciiHRTPostChkSum = cat(2,asciiHRTPreChkSum,asciiHRTChkSum,asciiMsgCRLF);

%%%%%%%%%%%%%%%%%%%%%%%%%%%%%%%%%%%%%%%%%%%%%%%%%%%%%%%%%%%%%%%%%%%%%

% Light tower message
asciiLITMsgID = uint8('$RXLIT,');

% Convert the light sequece into ascii code (1 = R, 2 = B, 3 = G)
asciiLITSeq = uint8(zeros(1,4)+32);
asciiLITSeq(4) = asciiMsgEnd;

if LITValid == 1
    for seqChar = 1:3
        if LITSequence(seqChar) == 1
            LITSequence(seqChar) = uint8('R');
        elseif LITSequence(seqChar) == 2
            LITSequence(seqChar) = uint8('B');
        elseif LITSequence(seqChar) == 3
            LITSequence(seqChar) = uint8('G');
        end
    end
    asciiLITSeq(1:3) = LITSequence;
end

% Concat individual ascii arrays into one array
asciiLITPreChkSum = cat(2,asciiLITMsgID,asciiTime,asciiTeamID,asciiLITSeq);

% Calculate the checksum of the message from the '$' to the '*' and convert
% to hex
LITchkSum = uint8(0);

for chksumChar = 1:(length(asciiLITPreChkSum)-2)
    LITchkSum = bitxor(LITchkSum,asciiLITPreChkSum(chksumChar+1));
end

% Convert the checksum to ascii
LITchkSum = dec2hex(LITchkSum);
asciiLITChkSum = uint8(zeros(1,length(LITchkSum))+32);
for i = 1:length(LITchkSum)
    asciiLITChkSum(i) = uint8(LITchkSum(i));
end

% Concat the checksum and the '/r/n' to the end of the message
asciiLITPostChkSum = cat(2,asciiLITPreChkSum,asciiLITChkSum,asciiMsgCRLF);

%%%%%%%%%%%%%%%%%%%%%%%%%%%%%%%%%%%%%%%%%%%%%%%%%%%%%%%%%%%%%%%%%%%%%%%%%%%

asciiHRTLITPostChkSum = cat(2,asciiHRTPostChkSum,asciiLITPostChkSum);
asciiHRTLIT(1:length(asciiHRTLITPostChkSum)) = asciiHRTLITPostChkSum;

== matlab function RobotX_ss_acousticsSingle_Dock_LB_1024/Main FSM/Start//Speedgate/Dead Reckon/Gate ==
  data: sglength input; ssHeldHeading input; Finished output; Valid output; X input; Y input; pts output
function [Finished, Valid, pts] = Gate(sglength,ssHeldHeading,X,Y)
%Written by Anderson Lebbad on August 9, 2014
%Last Edited by:

%This function sends a forward trajectory (from the initial heading read
%into it) until a landmark is found. Once the landmark is found, a
%trajectory is written to dodge around it.

pts = zeros(8,2);
Valid = 0;



persistent Found finPt
if isempty(Found)
    Found = 0;
    pts(1,1) = X + 5*cos(ssHeldHeading*pi/180);
    pts(1,2) = Y + 5*sin(ssHeldHeading*pi/180);
    pts(8,1) = X + sglength*cos(ssHeldHeading*pi/180);
    pts(8,2) = Y + sglength*sin(ssHeldHeading*pi/180);
    pts(2:7,:) = (1:6)'*(pts(8,:)-pts(1,:))/7+ones(6,1)*pts(1,:);
    Valid = 1;
    finPt = pts(8,:);
end

Finished = 0;

%Check to see how far the current pose is from the final point in the
%trajectory
range = abs(finPt(1)-X)+abs(finPt(2)-Y);


if range <= 10
    Finished = 1;
end

end

== matlab function RobotX_ss_acousticsSingle_Dock_LB_1024/Sensors/1024 Comms/Message Selector/HRTSEA Message/MATLAB Function ==
  data: Time input; HRTLat input; HRTLong input; HRTTask input; HRTMode input; SEAValid input; asciiHRTSEA output; SEALat input; SEALong input; SEAColor input; SEADepth input
function asciiHRTSEA = asciiHRTSEAEncoder(Time,HRTLat,HRTLong,HRTTask,HRTMode,SEAValid,SEALat,SEALong,SEAColor,SEADepth)

% Initialize output message vector as the serial output block expects 128
% character message
asciiHRTSEA = uint8(zeros(1,128));

asciiComma = uint8(',');
asciiDeciPt = uint8('.');
asciiTeamID = uint8('FAUVU,');
asciiMsgEnd = uint8('*');
asciiMsgCRLF = [13 10];

% Convert UTC Time input (hhmmss) into ascii code
asciiTime = uint8(zeros(1,7));
asciiTime(7) = asciiComma;

for timeChar = 1:6
    asciiTime(timeChar) = floor(mod(Time,10^(7-timeChar))/...
        10^(6-timeChar)) + 48;
end

%%%%%%%%%%%%%%%%%%%%%%%%%%%%%%%%%%%%%%%%%%%%%%%%%%%%%%%%%%%%%%%%%%%%
% Heartbeat message
% Convert static strings to ascii code
asciiHRTMsgID = uint8('$RXHRT,');
if HRTLat >= 0
    asciiHRTNS = uint8('N,');
else
    HRTLat = -HRTLat;
    asciiHRTNS = uint8('S,');
end
if HRTLong >= 0
    asciiHRTEW = uint8('E,');
else
    HRTLong = -HRTLong;
    asciiHRTEW = uint8('W,');
end

% Convert latitude (dd.mmmmmm) into ascii code
asciiHRTLat = uint8(zeros(1,10));
asciiHRTLat(10) = asciiComma;
asciiHRTLat(3) = asciiDeciPt;

HRTlatInt = floor(HRTLat);
for latIntChar = 1:2
    asciiHRTLat(latIntChar) = floor(mod(HRTlatInt,10^(3-latIntChar))/...
        10^(2-latIntChar)) + 48;
end

HRTlatDeci = mod(HRTLat,HRTlatInt) * 10^6;
for latDeciChar = 1:6
    asciiHRTLat(latDeciChar+3) = floor(mod(HRTlatDeci,10^(7-latDeciChar))/...
        10^(6-latDeciChar)) + 48;
end

% Convert longitude (ddd.mmmmmm) into ascii code
asciiHRTLong = uint8(zeros(1,11));
asciiHRTLong(11) = asciiComma;
asciiHRTLong(4) = asciiDeciPt;

HRTlongInt = floor(HRTLong);
for longIntChar = 1:3
    asciiHRTLong(longIntChar) = floor(mod(HRTlongInt,10^(4-longIntChar))/...
        10^(3-longIntChar)) + 48;
end

HRTlongDeci = mod(HRTLong,HRTlongInt) * 10^6;
for longDeciChar = 1:6
    asciiHRTLong(longDeciChar+4) = floor(mod(HRTlongDeci,10^(7-longDeciChar))/...
        10^(6-longDeciChar)) + 48;
end

% Convert vehicle mode into ascii (1 = RC, 2 = Auto)

% Auto On 
if HRTMode == 3 
    HRTOpMode = 2;
    asciiHRTMode = [uint8(HRTOpMode+48) asciiComma];
else
    HRTOpMode = 1;
    asciiHRTMode = [uint8(HRTOpMode+48) asciiComma];
end

% Convert vehicle task into ascii
HRTTask = HRTTask - 1; % FSM: Init = 1, SSGate = 2, SEA = 3, Dock = 4, LIT = 5, Obst = 6
if HRTTask ~= 1 || 2 || 3 || 4 || 5
    HRTOpTask = 1;
    asciiHRTTask = [uint8(HRTOpTask+48) asciiMsgEnd];
else
    asciiHRTTask = [uint8(HRTTask+48) asciiMsgEnd];
end

% Concat individual ascii arrays into one array
asciiHRTPreChkSum = cat(2,asciiHRTMsgID,asciiTime,asciiHRTLat,asciiHRTNS,asciiHRTLong,asciiHRTEW,...
    asciiTeamID,asciiHRTMode,asciiHRTTask);

% Calculate the checksum of the message from the '$' to the '*' and convert
% to hex
HRTchkSum = uint8(0);

for chksumChar = 1:(length(asciiHRTPreChkSum)-2)
    HRTchkSum = bitxor(HRTchkSum,asciiHRTPreChkSum(chksumChar+1));
end

% Convert the checksum to ascii
HRTchkSum = dec2hex(HRTchkSum);
asciiHRTChkSum = uint8(zeros(1,length(HRTchkSum))+32);
for i = 1:length(HRTchkSum)
    asciiHRTChkSum(i) = uint8(HRTchkSum(i));
end

% Concat the checksum and the '/r/n' to the end of the message
asciiHRTPostChkSum = cat(2,asciiHRTPreChkSum,asciiHRTChkSum,asciiMsgCRLF);

%%%%%%%%%%%%%%%%%%%%%%%%%%%%%%%%%%%%%%%%%%%%%%%%%%%%%%%%%%%%%%%%%%%%%

% Underwater search message
asciiSEAMsgID = uint8('$RXSEA,');
if SEAValid == 1
    if SEALat >= 0
        asciiSEANS = uint8('N,');
    else
        SEALat = -SEALat;
        asciiSEANS = uint8('S,');
    end
    if SEALong >= 0
        asciiSEAEW = uint8('E,');
    else
        SEALong = -SEALong;
        asciiSEAEW = uint8('W,');
    end
else
    asciiSEANS = [32 asciiComma];
    asciiSEAEW = [32 asciiComma];
end

% Convert buoy color to ascii code (1 = R, 2 = G, 3 = B, 4 = W, 5 = K)
asciiSEAColor = [uint8(32) asciiComma]; % Initialize as whitespace in case no buoy is found

if SEAColor == 1
    asciiSEAColor(1) = uint8('R');
elseif SEAColor == 2
    asciiSEAColor(1) = uint8('G');
elseif SEAColor == 3
    asciiSEAColor(1) = uint8('B');
elseif SEAColor == 4
    asciiSEAColor(1) = uint8('W');
elseif SEAColor == 5
    asciiSEAColor(1) = uint8('K');
end

% Convert latitude (dd.mmmmmm) into ascii code
asciiSEALat = uint8(zeros(1,10)+32); % Initialize as whitespace in case no buoy is found
asciiSEALat(10) = asciiComma;

% Only output values if valid bit is high
if SEAValid == 1
    asciiSEALat(3) = asciiDeciPt;
    SEAlatInt = floor(SEALat);
    for latIntChar = 1:2
        asciiSEALat(latIntChar) = floor(mod(SEAlatInt,10^(3-latIntChar))/...
            10^(2-latIntChar)) + 48;
    end
    
    SEAlatDeci = mod(SEALat,SEAlatInt) * 10^6;
    for latDeciChar = 1:6
        asciiSEALat(latDeciChar+3) = floor(mod(SEAlatDeci,10^(7-latDeciChar))/...
            10^(6-latDeciChar)) + 48;
    end
end

% Convert longitude (ddd.mmmmmm) into ascii code
asciiSEALong = uint8(zeros(1,11)+32); % Initialize as whitespace in case no buoy is found
asciiSEALong(11) = asciiComma;

% Only output values if valid bit is high
if SEAValid == 1
    asciiSEALong(4) = asciiDeciPt;
    SEAlongInt = floor(SEALong);
    for longIntChar = 1:3
        asciiSEALong(longIntChar) = floor(mod(SEAlongInt,10^(4-longIntChar))/...
            10^(3-longIntChar)) + 48;
    end
    
    SEAlongDeci = mod(SEALong,SEAlongInt) * 10^6;
    for longDeciChar = 1:6
        asciiSEALong(longDeciChar+4) = floor(mod(SEAlongDeci,10^(7-longDeciChar))/...
            10^(6-longDeciChar)) + 48;
    end
end

% Convert depth (m) (##.##) into ascii
asciiSEADepth = uint8(zeros(1,6)+32); % Initialize as whitespace in case no buoy is found
asciiSEADepth(6) = asciiMsgEnd;

% Only output values if valid bit is high
if SEAValid == 1
    asciiSEADepth(3) = asciiDeciPt;
    SEAdepthInt = floor(SEADepth);
    for depthIntChar = 1:2
        asciiSEADepth(depthIntChar) = floor(mod(SEAdepthInt,10^(3-depthIntChar))/...
            10^(2-depthIntChar)) + 48;
    end
    
    SEAdepthDeci = mod(SEADepth,SEAdepthInt) * 10^2;
    for depthDeciChar = 1:2
        asciiSEADepth(depthDeciChar+3) = floor(mod(SEAdepthDeci,10^(3-depthDeciChar))/...
            10^(2-depthDeciChar)) + 48;
    end
end

% Concat individual ascii arrays into one array
asciiSEAPreChkSum = cat(2,asciiSEAMsgID,asciiTime,asciiTeamID,asciiSEAColor,...
    asciiSEALat,asciiSEANS,asciiSEALong,asciiSEAEW,asciiSEADepth);

% Calculate the checksum of the message from the '$' to the '*' and convert
% to hex
SEAchkSum = uint8(0);

for chksumChar = 1:(length(asciiSEAPreChkSum)-2)
    SEAchkSum = bitxor(SEAchkSum,asciiSEAPreChkSum(chksumChar+1));
end

% Convert the checksum to ascii
SEAchkSum = dec2hex(SEAchkSum);
asciiSEAChkSum = uint8(zeros(1,length(SEAchkSum))+32);
for i = 1:length(SEAchkSum)
    asciiSEAChkSum(i) = uint8(SEAchkSum(i));
end

% Concat the checksum and the '/r/n' to the end of the message
asciiSEAPostChkSum = cat(2,asciiSEAPreChkSum,asciiSEAChkSum,asciiMsgCRLF);

%%%%%%%%%%%%%%%%%%%%%%%%%%%%%%%%%%%%%%%%%%%%%%%%%%%%%%%%%%%%%%%%%%%%%%

asciiHRTSEAPostChkSum = cat(2,asciiHRTPostChkSum,asciiSEAPostChkSum);
asciiHRTSEA(1:length(asciiHRTSEAPostChkSum)) = asciiHRTSEAPostChkSum;

== matlab function RobotX_ss_acousticsSingle_Dock_LB_1024/Main FSM/Start//Speedgate/Main Enabler ==
  data: taskSelector output; GpsEn output; entEn output; exitEn output; ssgateTask input; GpsFin input; entFin input
function [taskSelector,GpsEn,entEn,exitEn]=Startgate_Enabler(ssgateTask,...
    GpsFin,entFin)
%Written by Anderson Lebbad on July 19, 2013
%Last Edited: Dylan DeGaetano on September ,4 2014
%   Substring search for task was written in
%   Case switches were redundant, combined with first set of if statements

%Changes the value of MainMode and the enablers for the tasks within the
%Main FSM.

% Initialize enable signals
GpsEn = 0;
entEn =0;
exitEn = 0;

% Convert main task indicator to a string
ssgateTaskStr = char(ssgateTask);

% Adjust finished states based on user task selection (never skips
% initialization)
if ~isempty(strfind(ssgateTaskStr,'Aim'))
    GpsFin = 1;
elseif ~isempty(strfind(ssgateTaskStr,'Start'))
    GpsFin = 1;
    entFin = 1;
elseif ~isempty(strfind(ssgateTaskStr,'Speed'))
    GpsFin = 1;
    entFin = 1;
end

% Set enable signals based on state completion
if GpsFin == 0
    GpsEn = 1;
    taskSelector = 1;
elseif entFin == 0
    entEn = 1;
    taskSelector = 2;
else
    exitEn = 1;
    taskSelector = 3;
end

== matlab function RobotX_ss_acousticsSingle_Dock_LB_1024/Sensors/1024 Comms/Message Selector/HRTSEA Message/MATLAB Function1 ==
  data: pingerInfo input; SEAValid output; SEALat output; SEALong output; SEAColor output; SEADepth output
function [SEAValid,SEALat,SEALong,SEAColor,SEADepth] = pingerInfoParse(pingerInfo)

SEAValid = pingerInfo(1);
SEALat = pingerInfo(2);
SEALong = pingerInfo(3);
SEADepth = pingerInfo(4);
SEAColor = pingerInfo(5);

== matlab function RobotX_ss_acousticsSingle_Dock_LB_1024/Sensors/1024 Comms/Message Selector/HRTLIT Message/MATLAB Function1 ==
  data: ltSeq input; LITValid output; LITSequence output
function [LITValid,LITSequence] = LITSeqParse(ltSeq)

LITValid = ltSeq(1);
LITSequence = ltSeq(2:4);

== matlab function RobotX_ss_acousticsSingle_Dock_LB_1024/Sensors/1024 Comms/UTC Timer/MATLAB Function ==
  data: inTime input; timeOut output
function timeOut  = UTCtimer(inTime)
% This script works as a timer in UTC time (hhmmss) for the boat

persistent startTime

if isempty(startTime)
    startTime = inTime;
end

    hours = floor(startTime/10000);
    minutes = floor(mod(startTime,10000)/100);
    seconds = mod(startTime,100);
    
    if seconds > 59
        minutes = minutes + 1;
        seconds = 0;
    end
    
    if minutes > 59
        hours = hours + 1;
        minutes = 0;
    end
    
    if hours > 23
        hours = 0;
    end
    
    startTime = hours * 10000 + minutes * 100 + seconds;
    
    timeOut = floor(startTime);
    
    startTime = startTime + 0.25;
